simulink model "iir1"  (Simulink 6.1)
settings: Solver=FixedStepDiscrete  StartTime=0.0  StopTime=10.0  RelTol=1e-3
model workspace: external: M-Code (data not in the file)
undefined symbols (not defined in the file or in its folder): get
libraries: dspsigops x14, dspbuff3 x1, simulink x1, dspspect3 x1, dspsnks4 x1
settings Model: Creator=svenhoffmann  LastModifiedBy=svenhoffmann  ExtModeAutoUpdateStatusClock=off
settings DebuggingCC: SolverPrmCheckMsg=warning

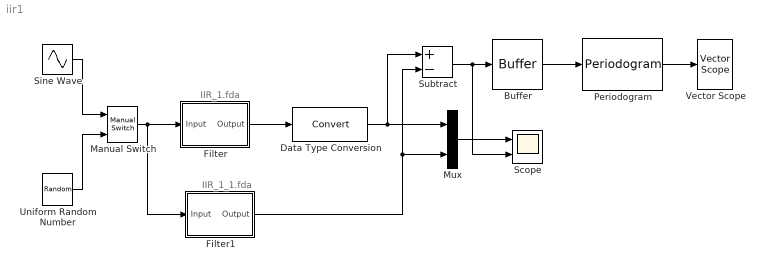
== system iir1 ==
  note: IIR_1_1.fda
  note: IIR_1.fda
  Buffer : dspbuff3/Buffer  N=256  V=64  ic=0
  Data Type Conversion : DataTypeConversion  OutDataTypeMode=double
  Filter : Subsystem  Tag=FilterWizardSubSystem
  Filter1 : Subsystem  Tag=FilterWizardSubSystem
  Manual Switch : simulink/Signal Routing/Manual Switch  sw=0  action=0
  Mux : Mux  Inputs=2
  Periodogram : dspspect3/Periodogram  wintype=Hamming  Rs=50  beta=5  winsamp=Symmetric  inheritFFT=off  fftsize=256  navg=4
  Scope : Scope  NumInputPorts=2
      settings: YMin=-5~-5  YMax=5~5
  Sine Wave : Sin  Amplitude=9.999694e-1  Frequency=2*pi*100  SampleTime=1/1000
  Subtract : Sum  Inputs=+-  OutScaling=2^-10
  Uniform Random Number : UniformRandomNumber  Minimum=-0.95  Maximum=0.95  SampleTime=1/1000
  Vector Scope : dspsnks4/Vector Scope  ScopeProperties=on  Domain=Frequency  HorizSpan=1  DisplayProperties=off  AxisGrid=on  Memory=off  FrameNumber=on  AxisLegend=off  AxisZoom=off  OpenScopeAtSimStart=on  OpenScopeImmediately=off  FigPos=get(0,'defaultfigureposition')  AxisProperties=off  XUnits=Hertz  XRange=[0...Fs/2]  InheritXIncr=off  XIncr=1/1000  XLabel=Time  YUnits=dB  YLabel=Amplitude  LineProperties=off
      settings: YMin=-106.145195657547  YMax=-75.386729288775
  wires:
  Filter/1(Output) -> Data Type Conversion/1
  Data Type Conversion/1 -> Mux/1, Subtract/1
  Mux/1 -> Scope/1
  Filter1/1(Output) -> Mux/2, Subtract/2
  Subtract/1 -> Buffer/1, Scope/2
  Periodogram/1 -> Vector Scope/1
  Buffer/1 -> Periodogram/1
  Manual Switch/1 -> Filter/1(Input), Filter1/1(Input)
  Sine Wave/1 -> Manual Switch/1
  Uniform Random Number/1 -> Manual Switch/2

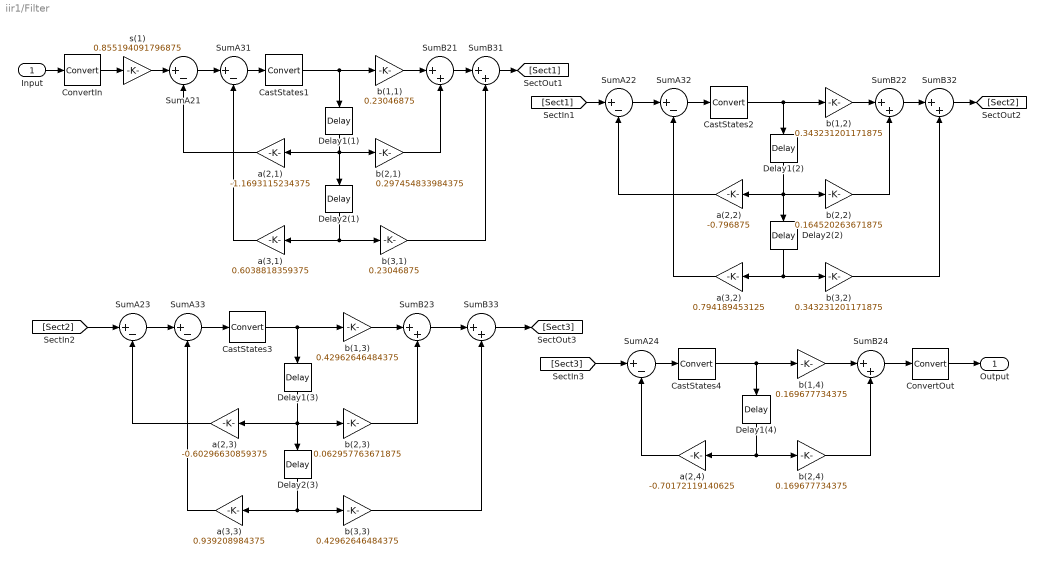
== system iir1/Filter ==
  Input : Inport  Port=1  LatchInput=off
  CastStates{1..4} (4 alike) : DataTypeConversion  OutDataTypeMode=Specify via dialog  OutDataType=sfix(18)  OutScaling=2^-14  RndMeth=Nearest  LockScale=on
  ConvertIn : DataTypeConversion  OutDataTypeMode=Specify via dialog  OutScaling=2^-15  RndMeth=Nearest  SaturateOnIntegerOverflow=on  LockScale=on
  ConvertOut : DataTypeConversion  OutDataTypeMode=Specify via dialog  OutScaling=2^-14  RndMeth=Nearest  LockScale=on
  Delay1(1) : dspsigops/Delay  Orientation=down  dly_unit=Samples  delay=1  ic_detail=off  dif_ic_for_ch=off  dif_ic_for_dly=off  ic=0  reset_popup=None
  Delay1(2) : dspsigops/Delay  Orientation=down  dly_unit=Samples  delay=1  ic_detail=off  dif_ic_for_ch=off  dif_ic_for_dly=off  ic=0  reset_popup=None
  Delay1(3) : dspsigops/Delay  Orientation=down  dly_unit=Samples  delay=1  ic_detail=off  dif_ic_for_ch=off  dif_ic_for_dly=off  ic=0  reset_popup=None
  Delay1(4) : dspsigops/Delay  Orientation=down  dly_unit=Samples  delay=1  ic_detail=off  dif_ic_for_ch=off  dif_ic_for_dly=off  ic=0  reset_popup=None
  Delay2(1) : dspsigops/Delay  Orientation=down  dly_unit=Samples  delay=1  ic_detail=off  dif_ic_for_ch=off  dif_ic_for_dly=off  ic=0  reset_popup=None
  Delay2(2) : dspsigops/Delay  Orientation=down  dly_unit=Samples  delay=1  ic_detail=off  dif_ic_for_ch=off  dif_ic_for_dly=off  ic=0  reset_popup=None
  Delay2(3) : dspsigops/Delay  Orientation=down  dly_unit=Samples  delay=1  ic_detail=off  dif_ic_for_ch=off  dif_ic_for_dly=off  ic=0  reset_popup=None
  SumA{21..24,31..33} (7 alike) : Sum  Inputs=|+-  OutDataTypeMode=Specify via dialog  OutDataType=sfix(40)  OutScaling=2^-26  RndMeth=Nearest  LockScale=on
  SumB{21..24,31..33} (7 alike) : Sum  Inputs=|++  OutDataTypeMode=Specify via dialog  OutDataType=sfix(40)  OutScaling=2^-27  RndMeth=Nearest  LockScale=on
  a(2,1) : Gain  Orientation=left  Gain=-1.1693115234375  ParameterDataTypeMode=Specify via dialog  ParameterScalingMode=Use specified scaling  ParameterScaling=2^-14  OutDataTypeMode=Specify via dialog  OutDataType=sfix(32)  OutScaling=2^-26  RndMeth=Nearest  LockScale=on
  a(2,2) : Gain  Orientation=left  Gain=-0.796875  ParameterDataTypeMode=Specify via dialog  ParameterScalingMode=Use specified scaling  ParameterScaling=2^-14  OutDataTypeMode=Specify via dialog  OutDataType=sfix(32)  OutScaling=2^-26  RndMeth=Nearest  LockScale=on
  a(2,3) : Gain  Orientation=left  Gain=-0.60296630859375  ParameterDataTypeMode=Specify via dialog  ParameterScalingMode=Use specified scaling  ParameterScaling=2^-14  OutDataTypeMode=Specify via dialog  OutDataType=sfix(32)  OutScaling=2^-26  RndMeth=Nearest  LockScale=on
  a(2,4) : Gain  Orientation=left  Gain=-0.70172119140625  ParameterDataTypeMode=Specify via dialog  ParameterScalingMode=Use specified scaling  ParameterScaling=2^-14  OutDataTypeMode=Specify via dialog  OutDataType=sfix(32)  OutScaling=2^-26  RndMeth=Nearest  LockScale=on
  a(3,1) : Gain  Orientation=left  Gain=0.6038818359375  ParameterDataTypeMode=Specify via dialog  ParameterScalingMode=Use specified scaling  ParameterScaling=2^-14  OutDataTypeMode=Specify via dialog  OutDataType=sfix(32)  OutScaling=2^-26  RndMeth=Nearest  LockScale=on
  a(3,2) : Gain  Orientation=left  Gain=0.794189453125  ParameterDataTypeMode=Specify via dialog  ParameterScalingMode=Use specified scaling  ParameterScaling=2^-14  OutDataTypeMode=Specify via dialog  OutDataType=sfix(32)  OutScaling=2^-26  RndMeth=Nearest  LockScale=on
  a(3,3) : Gain  Orientation=left  Gain=0.939208984375  ParameterDataTypeMode=Specify via dialog  ParameterScalingMode=Use specified scaling  ParameterScaling=2^-14  OutDataTypeMode=Specify via dialog  OutDataType=sfix(32)  OutScaling=2^-26  RndMeth=Nearest  LockScale=on
  b(1,1) : Gain  Gain=0.23046875  ParameterDataTypeMode=Specify via dialog  ParameterScalingMode=Use specified scaling  ParameterScaling=2^-15  OutDataTypeMode=Specify via dialog  OutDataType=sfix(32)  OutScaling=2^-27  RndMeth=Nearest  LockScale=on
  b(1,2) : Gain  Gain=0.343231201171875  ParameterDataTypeMode=Specify via dialog  ParameterScalingMode=Use specified scaling  ParameterScaling=2^-15  OutDataTypeMode=Specify via dialog  OutDataType=sfix(32)  OutScaling=2^-27  RndMeth=Nearest  LockScale=on
  b(1,3) : Gain  Gain=0.42962646484375  ParameterDataTypeMode=Specify via dialog  ParameterScalingMode=Use specified scaling  ParameterScaling=2^-15  OutDataTypeMode=Specify via dialog  OutDataType=sfix(32)  OutScaling=2^-27  RndMeth=Nearest  LockScale=on
  b(1,4) : Gain  Gain=0.169677734375  ParameterDataTypeMode=Specify via dialog  ParameterScalingMode=Use specified scaling  ParameterScaling=2^-15  OutDataTypeMode=Specify via dialog  OutDataType=sfix(32)  OutScaling=2^-27  RndMeth=Nearest  LockScale=on
  b(2,1) : Gain  Gain=0.297454833984375  ParameterDataTypeMode=Specify via dialog  ParameterScalingMode=Use specified scaling  ParameterScaling=2^-15  OutDataTypeMode=Specify via dialog  OutDataType=sfix(32)  OutScaling=2^-27  RndMeth=Nearest  LockScale=on
  b(2,2) : Gain  Gain=0.164520263671875  ParameterDataTypeMode=Specify via dialog  ParameterScalingMode=Use specified scaling  ParameterScaling=2^-15  OutDataTypeMode=Specify via dialog  OutDataType=sfix(32)  OutScaling=2^-27  RndMeth=Nearest  LockScale=on
  b(2,3) : Gain  Gain=0.062957763671875  ParameterDataTypeMode=Specify via dialog  ParameterScalingMode=Use specified scaling  ParameterScaling=2^-15  OutDataTypeMode=Specify via dialog  OutDataType=sfix(32)  OutScaling=2^-27  RndMeth=Nearest  LockScale=on
  b(2,4) : Gain  Gain=0.169677734375  ParameterDataTypeMode=Specify via dialog  ParameterScalingMode=Use specified scaling  ParameterScaling=2^-15  OutDataTypeMode=Specify via dialog  OutDataType=sfix(32)  OutScaling=2^-27  RndMeth=Nearest  LockScale=on
  b(3,1) : Gain  Gain=0.23046875  ParameterDataTypeMode=Specify via dialog  ParameterScalingMode=Use specified scaling  ParameterScaling=2^-15  OutDataTypeMode=Specify via dialog  OutDataType=sfix(32)  OutScaling=2^-27  RndMeth=Nearest  LockScale=on
  b(3,2) : Gain  Gain=0.343231201171875  ParameterDataTypeMode=Specify via dialog  ParameterScalingMode=Use specified scaling  ParameterScaling=2^-15  OutDataTypeMode=Specify via dialog  OutDataType=sfix(32)  OutScaling=2^-27  RndMeth=Nearest  LockScale=on
  b(3,3) : Gain  Gain=0.42962646484375  ParameterDataTypeMode=Specify via dialog  ParameterScalingMode=Use specified scaling  ParameterScaling=2^-15  OutDataTypeMode=Specify via dialog  OutDataType=sfix(32)  OutScaling=2^-27  RndMeth=Nearest  LockScale=on
  s(1) : Gain  Gain=0.855194091796875  ParameterDataTypeMode=Specify via dialog  ParameterScalingMode=Use specified scaling  ParameterScaling=2^-15  OutDataTypeMode=Specify via dialog  OutScaling=2^-14  RndMeth=Nearest  LockScale=on
  Output : Outport
  wires:
  Input/1 -> ConvertIn/1
  ConvertIn/1 -> s(1)/1
  s(1)/1 -> SumA21/1
  SumA21/1 -> SumA31/1
  SumA31/1 -> CastStates1/1
  CastStates1/1 -> b(1,1)/1, Delay1(1)/1
  b(1,1)/1 -> SumB21/1
  SumB21/1 -> SumB31/1
  SumB31/1 -> [Sect1]
  Delay1(1)/1 -> Delay2(1)/1, b(2,1)/1, a(2,1)/1
  b(2,1)/1 -> SumB21/2
  Delay2(1)/1 -> b(3,1)/1, a(3,1)/1
  b(3,1)/1 -> SumB31/2
  a(2,1)/1 -> SumA21/2
  a(3,1)/1 -> SumA31/2
  [Sect1] -> SumA22/1
  SumA22/1 -> SumA32/1
  SumA32/1 -> CastStates2/1
  CastStates2/1 -> b(1,2)/1, Delay1(2)/1
  b(1,2)/1 -> SumB22/1
  SumB22/1 -> SumB32/1
  SumB32/1 -> [Sect2]
  Delay1(2)/1 -> Delay2(2)/1, b(2,2)/1, a(2,2)/1
  b(2,2)/1 -> SumB22/2
  Delay2(2)/1 -> b(3,2)/1, a(3,2)/1
  b(3,2)/1 -> SumB32/2
  a(2,2)/1 -> SumA22/2
  a(3,2)/1 -> SumA32/2
  [Sect2] -> SumA23/1
  SumA23/1 -> SumA33/1
  SumA33/1 -> CastStates3/1
  CastStates3/1 -> b(1,3)/1, Delay1(3)/1
  b(1,3)/1 -> SumB23/1
  SumB23/1 -> SumB33/1
  SumB33/1 -> [Sect3]
  Delay1(3)/1 -> Delay2(3)/1, b(2,3)/1, a(2,3)/1
  b(2,3)/1 -> SumB23/2
  Delay2(3)/1 -> a(3,3)/1, b(3,3)/1
  b(3,3)/1 -> SumB33/2
  a(2,3)/1 -> SumA23/2
  a(3,3)/1 -> SumA33/2
  [Sect3] -> SumA24/1
  CastStates4/1 -> b(1,4)/1, Delay1(4)/1
  b(1,4)/1 -> SumB24/1
  ConvertOut/1 -> Output/1
  Delay1(4)/1 -> a(2,4)/1, b(2,4)/1
  b(2,4)/1 -> SumB24/2
  a(2,4)/1 -> SumA24/2
  SumB24/1 -> ConvertOut/1
  SumA24/1 -> CastStates4/1

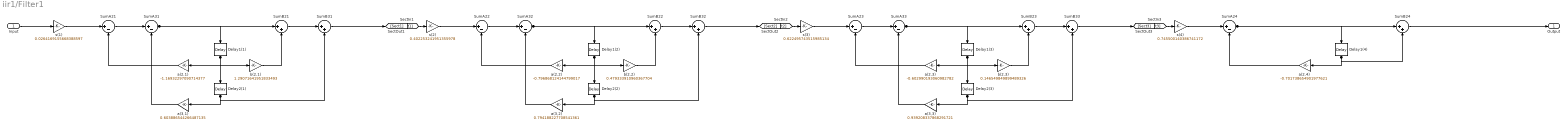
== system iir1/Filter1 ==
  Input : Inport  Port=1  LatchInput=off
  Delay1(1) : dspsigops/Delay  Orientation=down  dly_unit=Samples  delay=1  ic_detail=off  dif_ic_for_ch=off  dif_ic_for_dly=off  ic=0  reset_popup=None
  Delay1(2) : dspsigops/Delay  Orientation=down  dly_unit=Samples  delay=1  ic_detail=off  dif_ic_for_ch=off  dif_ic_for_dly=off  ic=0  reset_popup=None
  Delay1(3) : dspsigops/Delay  Orientation=down  dly_unit=Samples  delay=1  ic_detail=off  dif_ic_for_ch=off  dif_ic_for_dly=off  ic=0  reset_popup=None
  Delay1(4) : dspsigops/Delay  Orientation=down  dly_unit=Samples  delay=1  ic_detail=off  dif_ic_for_ch=off  dif_ic_for_dly=off  ic=0  reset_popup=None
  Delay2(1) : dspsigops/Delay  Orientation=down  dly_unit=Samples  delay=1  ic_detail=off  dif_ic_for_ch=off  dif_ic_for_dly=off  ic=0  reset_popup=None
  Delay2(2) : dspsigops/Delay  Orientation=down  dly_unit=Samples  delay=1  ic_detail=off  dif_ic_for_ch=off  dif_ic_for_dly=off  ic=0  reset_popup=None
  Delay2(3) : dspsigops/Delay  Orientation=down  dly_unit=Samples  delay=1  ic_detail=off  dif_ic_for_ch=off  dif_ic_for_dly=off  ic=0  reset_popup=None
  SumA{21..24,31..33} (7 alike) : Sum  Inputs=|+-  SaturateOnIntegerOverflow=on  InputSameDT=on
  SumB{21..24,31..33} (7 alike) : Sum  Inputs=|++  SaturateOnIntegerOverflow=on  InputSameDT=on
  a(2,1) : Gain  Orientation=left  Gain=-1.16932297090714377  SaturateOnIntegerOverflow=on
  a(2,2) : Gain  Orientation=left  Gain=-0.796868124144799017  SaturateOnIntegerOverflow=on
  a(2,3) : Gain  Orientation=left  Gain=-0.602990193060982782  SaturateOnIntegerOverflow=on
  a(2,4) : Gain  Orientation=left  Gain=-0.701738654901977621  SaturateOnIntegerOverflow=on
  a(3,1) : Gain  Orientation=left  Gain=0.603886544266487135  SaturateOnIntegerOverflow=on
  a(3,2) : Gain  Orientation=left  Gain=0.794188227708541361  SaturateOnIntegerOverflow=on
  a(3,3) : Gain  Orientation=left  Gain=0.939208337868291721  SaturateOnIntegerOverflow=on
  b(2,1) : Gain  Gain=1.29071641951833493  SaturateOnIntegerOverflow=on
  b(2,2) : Gain  Gain=0.479333910960367704  SaturateOnIntegerOverflow=on
  b(2,3) : Gain  Gain=0.146549849899489326  SaturateOnIntegerOverflow=on
  s(1) : Gain  Gain=0.0264169155668388597  SaturateOnIntegerOverflow=on
  s(2) : Gain  Gain=0.402253241951355978  SaturateOnIntegerOverflow=on
  s(3) : Gain  Gain=0.622495743515985134  SaturateOnIntegerOverflow=on
  s(4) : Gain  Gain=0.745500140386741172  SaturateOnIntegerOverflow=on
  Output : Outport
  wires:
  Input/1 -> s(1)/1
  s(1)/1 -> SumA21/1
  SumA21/1 -> SumA31/1
  SumA31/1 -> Delay1(1)/1, SumB21/1
  SumB21/1 -> SumB31/1
  SumB31/1 -> [Sect1]
  Delay1(1)/1 -> Delay2(1)/1, b(2,1)/1, a(2,1)/1
  b(2,1)/1 -> SumB21/2
  Delay2(1)/1 -> a(3,1)/1, SumB31/2
  a(2,1)/1 -> SumA21/2
  a(3,1)/1 -> SumA31/2
  [Sect1] -> s(2)/1
  s(2)/1 -> SumA22/1
  SumA22/1 -> SumA32/1
  SumA32/1 -> Delay1(2)/1, SumB22/1
  SumB22/1 -> SumB32/1
  SumB32/1 -> [Sect2]
  Delay1(2)/1 -> Delay2(2)/1, b(2,2)/1, a(2,2)/1
  b(2,2)/1 -> SumB22/2
  Delay2(2)/1 -> a(3,2)/1, SumB32/2
  a(2,2)/1 -> SumA22/2
  a(3,2)/1 -> SumA32/2
  [Sect2] -> s(3)/1
  s(3)/1 -> SumA23/1
  SumA23/1 -> SumA33/1
  SumA33/1 -> Delay1(3)/1, SumB23/1
  SumB23/1 -> SumB33/1
  SumB33/1 -> [Sect3]
  Delay1(3)/1 -> Delay2(3)/1, b(2,3)/1, a(2,3)/1
  b(2,3)/1 -> SumB23/2
  Delay2(3)/1 -> a(3,3)/1, SumB33/2
  a(2,3)/1 -> SumA23/2
  a(3,3)/1 -> SumA33/2
  [Sect3] -> s(4)/1
  s(4)/1 -> SumA24/1
  Delay1(4)/1 -> a(2,4)/1, SumB24/2
  a(2,4)/1 -> SumA24/2
  SumB24/1 -> Output/1
  SumA24/1 -> Delay1(4)/1, SumB24/1
